simulink model "Disc_ReducedOrder"  (R2021a)
settings: Solver=ode45  StartTime=0.0  StopTime=2  RelTol=1e-3
undefined symbols (not defined in the file): daq, digital_des_reduced, digital_des_reduced_int, DiscIntNeverNeededParam, drv, est_par, gbox, mot, rads2rpm, rpm2rads, sens, T_samp
settings Model: Creator=gioel  LastModifiedBy=gioel
settings DataIOCC: ReturnWorkspaceOutputs=off
settings DebuggingCC: AlgebraicLoopMsg=none

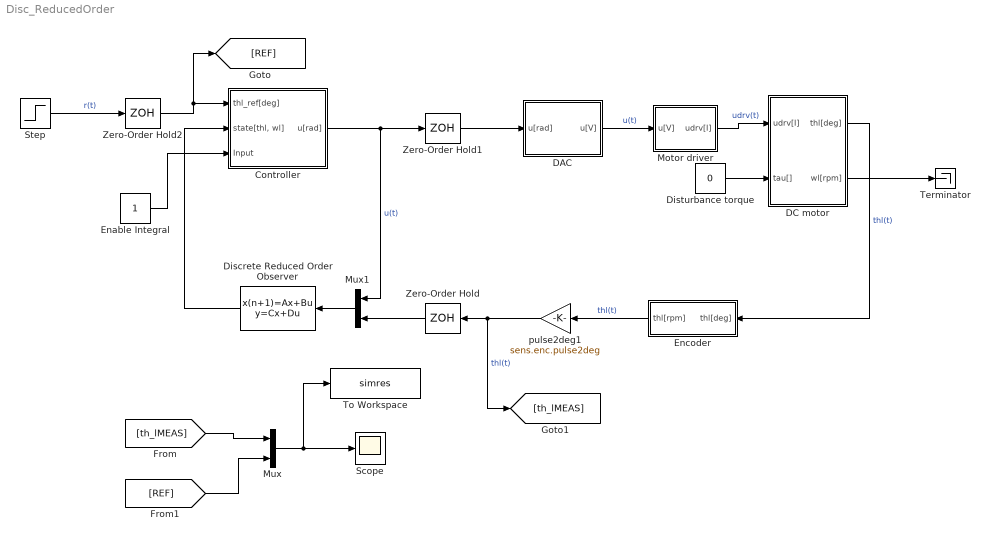
== system Disc_ReducedOrder ==
  Controller : Subsystem
  DAC : Subsystem
  DC motor : Subsystem
  Discrete Reduced Order Observer : DiscreteStateSpace  A=digital_des_reduced_int.Phy0  B=digital_des_reduced_int.Gamma0  C=digital_des_reduced_int.H0  D=digital_des_reduced_int.J0  SampleTime=T_samp
  Disturbance torque : Constant  Value=0
  Enable Integral : Constant
  Encoder : Subsystem
  Motor driver : Subsystem
  Mux : Mux  Inputs=2
  Mux1 : Mux  Inputs=2
  Scope : Scope
  Step : Step  Time=0  After=50  SampleTime=0
  Terminator : Terminator
  To Workspace : ToWorkspace  VariableName=simres  SaveFormat=Structure With Time  SampleTime=-1
  Zero-Order Hold : ZeroOrderHold  SampleTime=T_samp
  Zero-Order Hold1 : ZeroOrderHold  SampleTime=T_samp
  Zero-Order Hold2 : ZeroOrderHold  SampleTime=T_samp
  pulse2deg1 : Gain  Gain=sens.enc.pulse2deg
  wires:
  Zero-Order Hold1/1 -> DAC/1(u[rad])
  Zero-Order Hold/1 -> Mux1/2
  Mux1/1 -> Discrete Reduced Order Observer/1
  pulse2deg1/1 -> [th_lMEAS], Zero-Order Hold/1  "thl(t)"
  Step/1 -> Zero-Order Hold2/1  "r(t)"
  Zero-Order Hold2/1 -> Controller/1(thl_ref[deg]), [REF]
  DC motor/2(wl[rpm]) -> Terminator/1
  Encoder/1(thl[rpm]) -> pulse2deg1/1  "thl(t)"
  Motor driver/1(udrv[I]) -> DC motor/1(udrv[I])  "udrv(t)"
  DAC/1(u[V]) -> Motor driver/1(u[V])  "u(t)"
  DC motor/1(thl[deg]) -> Encoder/1(thl[deg])  "thl(t)"
  Disturbance torque/1 -> DC motor/2(tau[])
  Mux/1 -> To Workspace/1, Scope/1
  [th_lMEAS] -> Mux/1
  [REF] -> Mux/2
  Controller/1(u[rad]) -> Mux1/1, Zero-Order Hold1/1  "u(t)"
  Discrete Reduced Order Observer/1 -> Controller/2("state[thl, wl]")
  Enable Integral/1 -> Controller/3(Input)

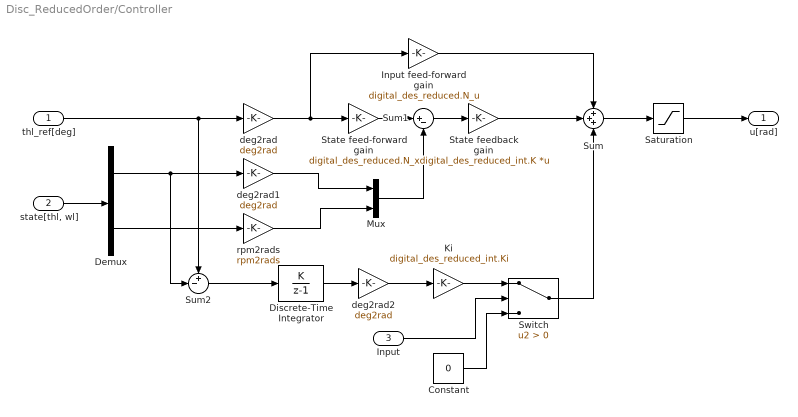
== system Disc_ReducedOrder/Controller ==
  thl_ref[deg] : Inport
  "state[thl, wl]" : Inport  Port=2
  Input : Inport  Port=3
  Constant : Constant  Value=0
  Demux : Demux  Outputs=2
  Discrete-Time Integrator : DiscreteIntegrator  IntegratorMethod=Accumulation: Forward Euler  SampleTime=T_samp  ICPrevOutput=DiscIntNeverNeededParam  ICPrevScaledInput=DiscIntNeverNeededParam
  Input feed-forward gain : Gain  Gain=digital_des_reduced.N_u
  Ki : Gain  Gain=digital_des_reduced_int.Ki
  Mux : Mux  Inputs=2
  Saturation : Saturate  UpperLimit=daq.dac.vdd  LowerLimit=daq.dac.vss
  State feed-forward gain : Gain  Gain=digital_des_reduced.N_x
  State feedback gain : Gain  Gain=digital_des_reduced_int.K  Multiplication=Matrix(K*u)
  Sum : Sum  Inputs=+++
  Sum1 : Sum  Inputs=|+-
  Sum2 : Sum  Inputs=+-|
  Switch : Switch  Criteria=u2 > Threshold
  deg2rad : Gain  Gain=deg2rad
  deg2rad1 : Gain  Gain=deg2rad
  deg2rad2 : Gain  Gain=deg2rad
  rpm2rads : Gain  Gain=rpm2rads
  u[rad] : Outport
  wires:
  rpm2rads/1 -> Mux/2
  Sum1/1 -> State feedback gain/1
  Mux/1 -> Sum1/2
  thl_ref[deg]/1 -> Sum2/1, deg2rad/1
  deg2rad/1 -> Input feed-forward gain/1, State feed-forward gain/1
  State feed-forward gain/1 -> Sum1/1
  deg2rad1/1 -> Mux/1
  Input feed-forward gain/1 -> Sum/1
  Saturation/1 -> u[rad]/1
  Demux/1 -> Sum2/2, deg2rad1/1
  State feedback gain/1 -> Sum/2
  Sum/1 -> Saturation/1
  Discrete-Time Integrator/1 -> deg2rad2/1
  deg2rad2/1 -> Ki/1
  Demux/2 -> rpm2rads/1
  "state[thl, wl]"/1 -> Demux/1
  Ki/1 -> Switch/1
  Switch/1 -> Sum/3
  Constant/1 -> Switch/3
  Input/1 -> Switch/2
  Sum2/1 -> Discrete-Time Integrator/1

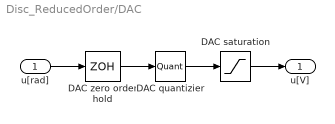
== system Disc_ReducedOrder/DAC ==
  u[rad] : Inport
  DAC quantizier : Quantizer  QuantizationInterval=daq.dac.q
  DAC saturation : Saturate  UpperLimit=10  LowerLimit=-10
  DAC zero order hold : ZeroOrderHold  SampleTime=sens.enc.T_s
  u[V] : Outport
  wires:
  DAC quantizier/1 -> DAC saturation/1
  DAC zero order hold/1 -> DAC quantizier/1
  DAC saturation/1 -> u[V]/1
  u[rad]/1 -> DAC zero order hold/1

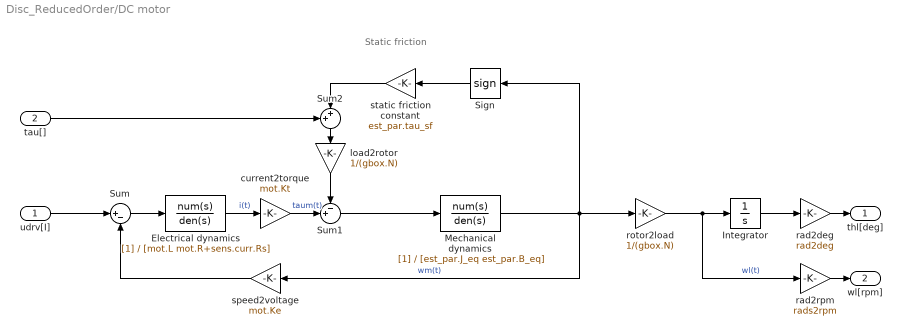
== system Disc_ReducedOrder/DC motor ==
  note: Static friction
  udrv[I] : Inport  Unit=V
  tau[] : Inport  Port=2  Unit=V
  Electrical dynamics : TransferFcn  Denominator=[mot.L mot.R+sens.curr.Rs]
  Integrator : Integrator
  Mechanical dynamics : TransferFcn  Denominator=[est_par.J_eq est_par.B_eq]
  Sign : Signum  ZeroCross=off
  Sum : Sum  Inputs=|+-
  Sum1 : Sum  Inputs=-+|
  Sum2 : Sum  Inputs=++|
  current2torque : Gain  Gain=mot.Kt
  load2rotor : Gain  Gain=1/(gbox.N)
  rad2deg : Gain  Gain=rad2deg
  rad2rpm : Gain  Gain=rads2rpm
  rotor2load : Gain  Gain=1/(gbox.N)
  speed2voltage : Gain  Gain=mot.Ke
  static friction constant : Gain  Gain=est_par.tau_sf
  thl[deg] : Outport  Unit=deg
  wl[rpm] : Outport  Port=2  Unit=rpm
  wires:
  load2rotor/1 -> Sum1/1
  Mechanical dynamics/1 -> Sign/1, rotor2load/1, speed2voltage/1  "wm(t)"
  Sign/1 -> static friction constant/1
  current2torque/1 -> Sum1/2  "taum(t)"
  Sum1/1 -> Mechanical dynamics/1
  speed2voltage/1 -> Sum/2
  rotor2load/1 -> rad2rpm/1, Integrator/1  "wl(t)"
  Electrical dynamics/1 -> current2torque/1  "i(t)"
  Integrator/1 -> rad2deg/1
  Sum/1 -> Electrical dynamics/1
  rad2rpm/1 -> wl[rpm]/1
  rad2deg/1 -> thl[deg]/1
  udrv[I]/1 -> Sum/1
  static friction constant/1 -> Sum2/2
  Sum2/1 -> load2rotor/1
  tau[]/1 -> Sum2/1

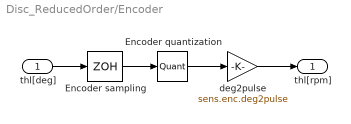
== system Disc_ReducedOrder/Encoder ==
  thl[deg] : Inport
  Encoder quantization : Quantizer  QuantizationInterval=sens.enc.q
  Encoder sampling : ZeroOrderHold  SampleTime=sens.enc.T_s
  deg2pulse : Gain  Gain=sens.enc.deg2pulse
  thl[rpm] : Outport
  wires:
  Encoder quantization/1 -> deg2pulse/1
  deg2pulse/1 -> thl[rpm]/1
  Encoder sampling/1 -> Encoder quantization/1
  thl[deg]/1 -> Encoder sampling/1

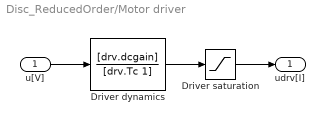
== system Disc_ReducedOrder/Motor driver ==
  u[V] : Inport
  Driver dynamics : TransferFcn  Numerator=[drv.dcgain]  Denominator=[drv.Tc 1]
  Driver saturation : Saturate  UpperLimit=12  LowerLimit=-12
  udrv[I] : Outport
  wires:
  Driver saturation/1 -> udrv[I]/1
  Driver dynamics/1 -> Driver saturation/1
  u[V]/1 -> Driver dynamics/1
